simulink library "halout"  (R2021b)
settings: Solver=VariableStepAuto  StartTime=0.0  StopTime=10.0  RelTol=1e-3
undefined symbols (not defined in the file): C_TASK_5MS_S, KHAL_CAN1TxReq_flg, KHAL_CAN2TxReq_flg, KHAL_CAN3TxReq_flg, KHAL_CAN4TxReq_flg, KHAL_CAN5TxReq_flg, KHAL_CAN6TxReq_flg, KHAL_CAN7TxReq_flg, TRUE
libraries: FVT_lib x65, simulink x6
(part 4 of 6)

== system halout/HAL_OUT/CAN7/FD7_C100_0_0x19F005D0 ==
  BSCP_outputs : Inport  OutDataTypeStr=Bus: BSCP_outputs
  BOUTP_outputs : Inport  Port=2  OutDataTypeStr=Bus: BOUTP_outputs
  VCUKeyStatus : Subsystem
  bus_creator : BusCreator  Inputs=1  OutDataTypeStr=Bus: DT_CAN7_SG_FD7_C100_0  NonVirtualBus=on
  bus_selector : BusSelector  OutputSignals=VOUTP_Keystatus_enum
  FD7_C100_0 : Outport
  wires:
  BSCP_outputs/1 -> [BSCP_outputs]
  BOUTP_outputs/1 -> [BOUTP_outputs]
  [CAN7_VCUKeyStatus] -> bus_creator/1  "CAN7_VCUKeyStatus"
  bus_creator/1 -> FD7_C100_0/1
  VCUKeyStatus/1(CAN7_VCUKeyStatus) -> [CAN7_VCUKeyStatus]
  bus_selector/1 -> VCUKeyStatus/1(VCUKeyStatus)  "<VOUTP_Keystatus_enum>"
  [BOUTP_outputs] -> bus_selector/1

== system halout/HAL_OUT/CAN7/FD7_C10_0_0xC61D0D1 ==
  BSCP_outputs : Inport  OutDataTypeStr=Bus: BSCP_outputs
  BOUTP_outputs : Inport  Port=2  OutDataTypeStr=Bus: BOUTP_outputs
  EMotorSpd : Subsystem
  bus_creator : BusCreator  Inputs=1  OutDataTypeStr=Bus: DT_CAN7_SG_FD7_C10_0  NonVirtualBus=on
  bus_selector : BusSelector  OutputSignals=VOUTP_EVCU1EMotorSpd_rpm
  FD7_C10_0 : Outport
  wires:
  BSCP_outputs/1 -> [BSCP_outputs]
  BOUTP_outputs/1 -> [BOUTP_outputs]
  [CAN7_EMotorSpd] -> bus_creator/1  "CAN7_EMotorSpd"
  bus_creator/1 -> FD7_C10_0/1
  EMotorSpd/1(CAN7_EMotorSpd) -> [CAN7_EMotorSpd]
  bus_selector/1 -> EMotorSpd/1(EMotorSpd)  "<VOUTP_EVCU1EMotorSpd_rpm>"
  [BOUTP_outputs] -> bus_selector/1

== system halout/HAL_OUT/CAN7/FD7_C200_0_0x18F003EF ==
  BSCP_outputs : Inport  OutDataTypeStr=Bus: BSCP_outputs
  BOUTP_outputs : Inport  Port=2  OutDataTypeStr=Bus: BOUTP_outputs
  SysPowerMode : Subsystem
  bus_creator : BusCreator  Inputs=1  OutDataTypeStr=Bus: DT_CAN7_SG_FD7_C200_0  NonVirtualBus=on
  bus_selector : BusSelector  OutputSignals=VOUTP_SysPowerMode_enum
  FD7_C200_0 : Outport
  wires:
  BSCP_outputs/1 -> [BSCP_outputs]
  BOUTP_outputs/1 -> [BOUTP_outputs]
  [CAN7_SysPowerMode] -> bus_creator/1  "CAN7_SysPowerMode"
  bus_creator/1 -> FD7_C200_0/1
  SysPowerMode/1(CAN7_SysPowerMode) -> [CAN7_SysPowerMode]
  bus_selector/1 -> SysPowerMode/1(SysPowerMode)  "<VOUTP_SysPowerMode_enum>"
  [BOUTP_outputs] -> bus_selector/1

== system halout/HAL_OUT/CAN7/FD7_C50_0_0xCF00300 ==
  BSCP_outputs : Inport  OutDataTypeStr=Bus: BSCP_outputs
  BOUTP_outputs : Inport  Port=2  OutDataTypeStr=Bus: BOUTP_outputs
  AccPedalPos1 : Subsystem
  Ground : Ground
  bus_creator : BusCreator  Inputs=1  OutDataTypeStr=Bus: DT_CAN7_SG_FD7_C50_0  NonVirtualBus=on
  FD7_C50_0 : Outport
  wires:
  BSCP_outputs/1 -> [BSCP_outputs]
  BOUTP_outputs/1 -> [BOUTP_outputs]
  [CAN7_AccPedalPos1] -> bus_creator/1  "CAN7_AccPedalPos1"
  bus_creator/1 -> FD7_C50_0/1
  AccPedalPos1/1(CAN7_AccPedalPos1) -> [CAN7_AccPedalPos1]
  Ground/1 -> AccPedalPos1/1(AccPedalPos1)

== system halout/HAL_OUT/CAN7/FD7_CE100_0_0x18FA05B9 ==
  BSCP_outputs : Inport  OutDataTypeStr=Bus: BSCP_outputs
  BOUTP_outputs : Inport  Port=2  OutDataTypeStr=Bus: BOUTP_outputs
  FDCBCMDVRSignalLCmd : Subsystem
  FDCBCMDVRSignalRCmd : Subsystem
  FDCBCMFDoorSta : Subsystem
  FDCBCMHBeamCmd : Subsystem
  FDCBCMLBeamCmd : Subsystem
  FDCBCMMDoorSta : Subsystem
  FDCBCMPLampCmd : Subsystem
  bus_creator : BusCreator  Inputs=7  OutDataTypeStr=Bus: DT_CAN7_SG_FD7_CE100_0  NonVirtualBus=on
  bus_selector : BusSelector  OutputSignals=VOUTP_FDCBCMDVRSignalLCmd_flg
  bus_selector1 : BusSelector  OutputSignals=VOUTP_FDCBCMDVRSignalRCmd_flg
  bus_selector2 : BusSelector  OutputSignals=VOUTP_FDCBCMFDoorSta_flg
  bus_selector3 : BusSelector  OutputSignals=VOUTP_FDCBCMHBeamCmd_flg
  bus_selector4 : BusSelector  OutputSignals=VOUTP_FDCBCMLBeamCmd_flg
  bus_selector5 : BusSelector  OutputSignals=VOUTP_FDCBCMMDoorSta_flg
  bus_selector6 : BusSelector  OutputSignals=VOUTP_FDCBCMPLampCmd_flg
  FD7_CE100_0 : Outport
  wires:
  BSCP_outputs/1 -> [BSCP_outputs]
  BOUTP_outputs/1 -> [BOUTP_outputs]
  [CAN7_FDC_BCM_DVRSignalL_Cmd] -> bus_creator/1  "CAN7_FDC_BCM_DVRSignalL_Cmd"
  [CAN7_FDC_BCM_DVRSignalR_Cmd] -> bus_creator/2  "CAN7_FDC_BCM_DVRSignalR_Cmd"
  [CAN7_FDC_BCM_FDoor_Sta] -> bus_creator/3  "CAN7_FDC_BCM_FDoor_Sta"
  [CAN7_FDC_BCM_HBeam_Cmd] -> bus_creator/4  "CAN7_FDC_BCM_HBeam_Cmd"
  [CAN7_FDC_BCM_LBeam_Cmd] -> bus_creator/5  "CAN7_FDC_BCM_LBeam_Cmd"
  [CAN7_FDC_BCM_MDoor_Sta] -> bus_creator/6  "CAN7_FDC_BCM_MDoor_Sta"
  [CAN7_FDC_BCM_PLamp_Cmd] -> bus_creator/7  "CAN7_FDC_BCM_PLamp_Cmd"
  bus_creator/1 -> FD7_CE100_0/1
  FDCBCMDVRSignalLCmd/1(CAN7_FDC_BCM_DVRSignalL_Cmd) -> [CAN7_FDC_BCM_DVRSignalL_Cmd]
  FDCBCMDVRSignalRCmd/1(CAN7_FDC_BCM_DVRSignalR_Cmd) -> [CAN7_FDC_BCM_DVRSignalR_Cmd]
  FDCBCMFDoorSta/1(CAN7_FDC_BCM_FDoor_Sta) -> [CAN7_FDC_BCM_FDoor_Sta]
  FDCBCMHBeamCmd/1(CAN7_FDC_BCM_HBeam_Cmd) -> [CAN7_FDC_BCM_HBeam_Cmd]
  FDCBCMLBeamCmd/1(CAN7_FDC_BCM_LBeam_Cmd) -> [CAN7_FDC_BCM_LBeam_Cmd]
  FDCBCMMDoorSta/1(CAN7_FDC_BCM_MDoor_Sta) -> [CAN7_FDC_BCM_MDoor_Sta]
  FDCBCMPLampCmd/1(CAN7_FDC_BCM_PLamp_Cmd) -> [CAN7_FDC_BCM_PLamp_Cmd]
  bus_selector/1 -> FDCBCMDVRSignalLCmd/1(FDCBCMDVRSignalLCmd)  "<VOUTP_FDCBCMDVRSignalLCmd_flg>"
  [BOUTP_outputs] -> bus_selector/1
  bus_selector1/1 -> FDCBCMDVRSignalRCmd/1(FDCBCMDVRSignalRCmd)  "<VOUTP_FDCBCMDVRSignalRCmd_flg>"
  [BOUTP_outputs] -> bus_selector1/1
  bus_selector2/1 -> FDCBCMFDoorSta/1(FDCBCMFDoorSta)  "<VOUTP_FDCBCMFDoorSta_flg>"
  [BOUTP_outputs] -> bus_selector2/1
  bus_selector3/1 -> FDCBCMHBeamCmd/1(FDCBCMHBeamCmd)  "<VOUTP_FDCBCMHBeamCmd_flg>"
  [BOUTP_outputs] -> bus_selector3/1
  bus_selector4/1 -> FDCBCMLBeamCmd/1(FDCBCMLBeamCmd)  "<VOUTP_FDCBCMLBeamCmd_flg>"
  [BOUTP_outputs] -> bus_selector4/1
  bus_selector5/1 -> FDCBCMMDoorSta/1(FDCBCMMDoorSta)  "<VOUTP_FDCBCMMDoorSta_flg>"
  [BOUTP_outputs] -> bus_selector5/1
  bus_selector6/1 -> FDCBCMPLampCmd/1(FDCBCMPLampCmd)  "<VOUTP_FDCBCMPLampCmd_flg>"
  [BOUTP_outputs] -> bus_selector6/1

== system halout/HAL_OUT/CAN1/FD1_C100_0_0x18FE4A03/VCUEBSRd4BR ==
  VCUEBSRd4BR : Inport
  Data Type Conversion : DataTypeConversion  OutDataTypeStr=uint8  RndMeth=Round
  CAN1_VCUEBSRd4BR : Outport
  wires:
  Data Type Conversion/1 -> CAN1_VCUEBSRd4BR/1
  VCUEBSRd4BR/1 -> Data Type Conversion/1

== system halout/HAL_OUT/CAN1/FD1_C100_1_0x18FF602B/VCUEBSHBSw ==
  VCUEBSHBSw : Inport
  Data Type Conversion : DataTypeConversion  OutDataTypeStr=uint8  RndMeth=Round
  CAN1_VCUEBSHBSw : Outport
  wires:
  Data Type Conversion/1 -> CAN1_VCUEBSHBSw/1
  VCUEBSHBSw/1 -> Data Type Conversion/1

== system halout/HAL_OUT/CAN1/FD1_C100_1_0x18FF602B/VCUEBSHHSw ==
  VCUEBSHHSw : Inport
  Data Type Conversion : DataTypeConversion  OutDataTypeStr=uint8  RndMeth=Round
  CAN1_VCUEBSHHSw : Outport
  wires:
  Data Type Conversion/1 -> CAN1_VCUEBSHHSw/1
  VCUEBSHHSw/1 -> Data Type Conversion/1

== system halout/HAL_OUT/CAN1/FD1_C100_2_0x19F005D0/GearFlashInd ==
  GearFlashInd : Inport
  Data Type Conversion : DataTypeConversion  OutDataTypeStr=uint8  RndMeth=Round
  CAN1_GearFlashInd : Outport
  wires:
  Data Type Conversion/1 -> CAN1_GearFlashInd/1
  GearFlashInd/1 -> Data Type Conversion/1

== system halout/HAL_OUT/CAN1/FD1_C100_2_0x19F005D0/LVBattLow ==
  LVBattLow : Inport
  Data Type Conversion : DataTypeConversion  OutDataTypeStr=uint8  RndMeth=Round
  CAN1_LVBattLow : Outport
  wires:
  Data Type Conversion/1 -> CAN1_LVBattLow/1
  LVBattLow/1 -> Data Type Conversion/1

== system halout/HAL_OUT/CAN1/FD1_C100_2_0x19F005D0/PweLmtInd ==
  PweLmtInd : Inport
  Data Type Conversion : DataTypeConversion  OutDataTypeStr=uint8  RndMeth=Round
  CAN1_PweLmtInd : Outport
  wires:
  Data Type Conversion/1 -> CAN1_PweLmtInd/1
  PweLmtInd/1 -> Data Type Conversion/1

== system halout/HAL_OUT/CAN1/FD1_C100_2_0x19F005D0/VCUBCMBuzzReq ==
  VCUBCMBuzzReq : Inport
  Data Type Conversion : DataTypeConversion  OutDataTypeStr=uint8  RndMeth=Round
  CAN1_VCUBCMBuzzReq : Outport
  wires:
  Data Type Conversion/1 -> CAN1_VCUBCMBuzzReq/1
  VCUBCMBuzzReq/1 -> Data Type Conversion/1

== system halout/HAL_OUT/CAN1/FD1_C100_2_0x19F005D0/VCUDTCCurrCode ==
  VCUDTCCurrCode : Inport
  Data Type Conversion : DataTypeConversion  OutDataTypeStr=uint32  RndMeth=Round
  CAN1_VCUDTCCurrCode : Outport
  wires:
  Data Type Conversion/1 -> CAN1_VCUDTCCurrCode/1
  VCUDTCCurrCode/1 -> Data Type Conversion/1

== system halout/HAL_OUT/CAN1/FD1_C100_2_0x19F005D0/VCUDTCCurrSta ==
  VCUDTCCurrSta : Inport
  Data Type Conversion : DataTypeConversion  OutDataTypeStr=uint8  RndMeth=Round
  CAN1_VCUDTCCurrSta : Outport
  wires:
  Data Type Conversion/1 -> CAN1_VCUDTCCurrSta/1
  VCUDTCCurrSta/1 -> Data Type Conversion/1

== system halout/HAL_OUT/CAN1/FD1_C100_2_0x19F005D0/VCUDTCHisCode ==
  VCUDTCHisCode : Inport
  Data Type Conversion : DataTypeConversion  OutDataTypeStr=uint32  RndMeth=Round
  CAN1_VCUDTCHisCode : Outport
  wires:
  Data Type Conversion/1 -> CAN1_VCUDTCHisCode/1
  VCUDTCHisCode/1 -> Data Type Conversion/1

== system halout/HAL_OUT/CAN1/FD1_C100_2_0x19F005D0/VCUDTCHisSta ==
  VCUDTCHisSta : Inport
  Data Type Conversion : DataTypeConversion  OutDataTypeStr=uint8  RndMeth=Round
  CAN1_VCUDTCHisSta : Outport
  wires:
  Data Type Conversion/1 -> CAN1_VCUDTCHisSta/1
  VCUDTCHisSta/1 -> Data Type Conversion/1

== system halout/HAL_OUT/CAN1/FD1_C100_2_0x19F005D0/VCUKeyStatus ==
  VCUKeyStatus : Inport
  Data Type Conversion : DataTypeConversion  OutDataTypeStr=uint8  RndMeth=Round
  CAN1_VCUKeyStatus : Outport
  wires:
  Data Type Conversion/1 -> CAN1_VCUKeyStatus/1
  VCUKeyStatus/1 -> Data Type Conversion/1

== system halout/HAL_OUT/CAN1/FD1_C100_2_0x19F005D0/VCUWarnInd ==
  VCUWarnInd : Inport
  Data Type Conversion : DataTypeConversion  OutDataTypeStr=uint8  RndMeth=Round
  CAN1_VCUWarnInd : Outport
  wires:
  Data Type Conversion/1 -> CAN1_VCUWarnInd/1
  VCUWarnInd/1 -> Data Type Conversion/1

== system halout/HAL_OUT/CAN1/FD1_C100_2_0x19F005D0/VCUnoPBInd ==
  VCUnoPBInd : Inport
  Data Type Conversion : DataTypeConversion  OutDataTypeStr=uint8  RndMeth=Round
  CAN1_VCUnoPBInd : Outport
  wires:
  Data Type Conversion/1 -> CAN1_VCUnoPBInd/1
  VCUnoPBInd/1 -> Data Type Conversion/1

== system halout/HAL_OUT/CAN1/FD1_C100_3_0x18FEF100/BrakeSW ==
  BrakeSW : Inport
  Data Type Conversion : DataTypeConversion  OutDataTypeStr=uint8  RndMeth=Round
  CAN1_BrakeSW : Outport
  wires:
  Data Type Conversion/1 -> CAN1_BrakeSW/1
  BrakeSW/1 -> Data Type Conversion/1

== system halout/HAL_OUT/CAN1/FD1_C100_3_0x18FEF100/VCUVehSpd ==
  VCUVehSpd : Inport
  Data Type Conversion : DataTypeConversion  OutDataTypeStr=uint16  RndMeth=Round
  convert_out : FVT_lib/hal/convert_out  gain=0.00391  offset=0
  CAN1_VCUVehSpd : Outport
  wires:
  Data Type Conversion/1 -> CAN1_VCUVehSpd/1
  convert_out/1 -> Data Type Conversion/1
  VCUVehSpd/1 -> convert_out/1

== system halout/HAL_OUT/CAN1/FD1_C10_0_0xC61D0D1/VehActDriveDirect ==
  VehActDriveDirect : Inport
  Data Type Conversion : DataTypeConversion  OutDataTypeStr=uint8  RndMeth=Round
  CAN1_VehActDriveDirect : Outport
  wires:
  Data Type Conversion/1 -> CAN1_VehActDriveDirect/1
  VehActDriveDirect/1 -> Data Type Conversion/1

== system halout/HAL_OUT/CAN1/FD1_C10_1_0x18FF20EF/ActEMOutSftSpd ==
  ActEMOutSftSpd : Inport
  Data Type Conversion : DataTypeConversion  OutDataTypeStr=uint16  RndMeth=Round
  convert_out : FVT_lib/hal/convert_out  gain=0.25  offset=0
  CAN1_ActEMOutSftSpd : Outport
  wires:
  Data Type Conversion/1 -> CAN1_ActEMOutSftSpd/1
  convert_out/1 -> Data Type Conversion/1
  ActEMOutSftSpd/1 -> convert_out/1

== system halout/HAL_OUT/CAN1/FD1_C10_1_0x18FF20EF/ActEMpTrq ==
  ActEMpTrq : Inport
  Data Type Conversion : DataTypeConversion  OutDataTypeStr=uint8  RndMeth=Round
  convert_out : FVT_lib/hal/convert_out  gain=1  offset=-125
  CAN1_ActEMpTrq : Outport
  wires:
  Data Type Conversion/1 -> CAN1_ActEMpTrq/1
  convert_out/1 -> Data Type Conversion/1
  ActEMpTrq/1 -> convert_out/1

== system halout/HAL_OUT/CAN1/FD1_C10_1_0x18FF20EF/ActEMpTrqHrls ==
  ActEMpTrqHrls : Inport
  Data Type Conversion : DataTypeConversion  OutDataTypeStr=uint8  RndMeth=Round
  convert_out : FVT_lib/hal/convert_out  gain=0.125  offset=0
  CAN1_ActEMpTrqHrls : Outport
  wires:
  Data Type Conversion/1 -> CAN1_ActEMpTrqHrls/1
  convert_out/1 -> Data Type Conversion/1
  ActEMpTrqHrls/1 -> convert_out/1

== system halout/HAL_OUT/CAN1/FD1_C10_1_0x18FF20EF/ActMaxAvaEMRecpTrq ==
  ActMaxAvaEMRecpTrq : Inport
  Data Type Conversion : DataTypeConversion  OutDataTypeStr=uint8  RndMeth=Round
  convert_out : FVT_lib/hal/convert_out  gain=1  offset=-125
  CAN1_ActMaxAvaEMRecpTrq : Outport
  wires:
  Data Type Conversion/1 -> CAN1_ActMaxAvaEMRecpTrq/1
  convert_out/1 -> Data Type Conversion/1
  ActMaxAvaEMRecpTrq/1 -> convert_out/1

== system halout/HAL_OUT/CAN1/FD1_C10_1_0x18FF20EF/DrvDemEMRtapTrq ==
  DrvDemEMRtapTrq : Inport
  Data Type Conversion : DataTypeConversion  OutDataTypeStr=uint8  RndMeth=Round
  convert_out : FVT_lib/hal/convert_out  gain=1  offset=-125
  CAN1_DrvDemEMRtapTrq : Outport
  wires:
  Data Type Conversion/1 -> CAN1_DrvDemEMRtapTrq/1
  convert_out/1 -> Data Type Conversion/1
  DrvDemEMRtapTrq/1 -> convert_out/1

== system halout/HAL_OUT/CAN1/FD1_C10_1_0x18FF20EF/EMTrqModeDrvBrk ==
  EMTrqModeDrvBrk : Inport
  Data Type Conversion : DataTypeConversion  OutDataTypeStr=uint8  RndMeth=Round
  CAN1_EMTrqModeDrvBrk : Outport
  wires:
  Data Type Conversion/1 -> CAN1_EMTrqModeDrvBrk/1
  EMTrqModeDrvBrk/1 -> Data Type Conversion/1

== system halout/HAL_OUT/CAN1/FD1_C10_1_0x18FF20EF/RetSelNonEng ==
  RetSelNonEng : Inport
  Data Type Conversion : DataTypeConversion  OutDataTypeStr=uint8  RndMeth=Round
  convert_out : FVT_lib/hal/convert_out  gain=0.4  offset=0
  CAN1_RetSelNonEng : Outport
  wires:
  Data Type Conversion/1 -> CAN1_RetSelNonEng/1
  convert_out/1 -> Data Type Conversion/1
  RetSelNonEng/1 -> convert_out/1

== system halout/HAL_OUT/CAN1/FD1_C10_1_0x18FF20EF/SACtrlDev ==
  SACtrlDev : Inport
  Data Type Conversion : DataTypeConversion  OutDataTypeStr=uint8  RndMeth=Round
  CAN1_SACtrlDev : Outport
  wires:
  Data Type Conversion/1 -> CAN1_SACtrlDev/1
  SACtrlDev/1 -> Data Type Conversion/1

== system halout/HAL_OUT/CAN1/FD1_C200_0_0x18F003EF/SysPowerMode ==
  SysPowerMode : Inport
  Data Type Conversion : DataTypeConversion  OutDataTypeStr=uint8  RndMeth=Round
  CAN1_SysPowerMode : Outport
  wires:
  Data Type Conversion/1 -> CAN1_SysPowerMode/1
  SysPowerMode/1 -> Data Type Conversion/1

== system halout/HAL_OUT/CAN1/FD1_C20_0_0xC62D0D1/DCCurr ==
  DCCurr : Inport
  Data Type Conversion : DataTypeConversion  OutDataTypeStr=uint16  RndMeth=Round
  convert_out : FVT_lib/hal/convert_out  gain=0.05  offset=-1638.4
  CAN1_DCCurr : Outport
  wires:
  Data Type Conversion/1 -> CAN1_DCCurr/1
  convert_out/1 -> Data Type Conversion/1
  DCCurr/1 -> convert_out/1

== system halout/HAL_OUT/CAN1/FD1_C20_0_0xC62D0D1/DCVol ==
  DCVol : Inport
  Data Type Conversion : DataTypeConversion  OutDataTypeStr=uint16  RndMeth=Round
  convert_out : FVT_lib/hal/convert_out  gain=0.25  offset=0
  CAN1_DCVol : Outport
  wires:
  Data Type Conversion/1 -> CAN1_DCVol/1
  convert_out/1 -> Data Type Conversion/1
  DCVol/1 -> convert_out/1

== system halout/HAL_OUT/CAN1/FD1_C20_0_0xC62D0D1/MaxTorqAvail ==
  MaxTorqAvail : Inport
  Data Type Conversion : DataTypeConversion  OutDataTypeStr=uint16  RndMeth=Round
  convert_out : FVT_lib/hal/convert_out  gain=1  offset=-125
  CAN1_MaxTorqAvail : Outport
  wires:
  Data Type Conversion/1 -> CAN1_MaxTorqAvail/1
  convert_out/1 -> Data Type Conversion/1
  MaxTorqAvail/1 -> convert_out/1

== system halout/HAL_OUT/CAN1/FD1_C20_0_0xC62D0D1/MinTorqAvail ==
  MinTorqAvail : Inport
  Data Type Conversion : DataTypeConversion  OutDataTypeStr=uint16  RndMeth=Round
  convert_out : FVT_lib/hal/convert_out  gain=1  offset=-125
  CAN1_MinTorqAvail : Outport
  wires:
  Data Type Conversion/1 -> CAN1_MinTorqAvail/1
  convert_out/1 -> Data Type Conversion/1
  MinTorqAvail/1 -> convert_out/1

== system halout/HAL_OUT/CAN1/FD1_C250_0_0x18FEDFEF/EMParasLoss ==
  EMParasLoss : Inport
  Data Type Conversion : DataTypeConversion  OutDataTypeStr=uint8  RndMeth=Round
  convert_out : FVT_lib/hal/convert_out  gain=1  offset=-125
  CAN1_EMParasLoss : Outport
  wires:
  Data Type Conversion/1 -> CAN1_EMParasLoss/1
  convert_out/1 -> Data Type Conversion/1
  EMParasLoss/1 -> convert_out/1

== system halout/HAL_OUT/CAN1/FD1_C250_0_0x18FEDFEF/NFricPercTorq ==
  NFricPercTorq : Inport
  Data Type Conversion : DataTypeConversion  OutDataTypeStr=uint8  RndMeth=Round
  convert_out : FVT_lib/hal/convert_out  gain=1  offset=-125
  CAN1_NFricPercTorq : Outport
  wires:
  Data Type Conversion/1 -> CAN1_NFricPercTorq/1
  convert_out/1 -> Data Type Conversion/1
  NFricPercTorq/1 -> convert_out/1

== system halout/HAL_OUT/CAN1/FD1_C5000_0_0x18FEE1EF/RC1MaxRetSpdP2 ==
  RC1MaxRetSpdP2 : Inport
  Data Type Conversion : DataTypeConversion  OutDataTypeStr=uint16  RndMeth=Round
  convert_out : FVT_lib/hal/convert_out  gain=0.125  offset=0
  CAN1_RC1MaxRetSpdP2 : Outport
  wires:
  Data Type Conversion/1 -> CAN1_RC1MaxRetSpdP2/1
  convert_out/1 -> Data Type Conversion/1
  RC1MaxRetSpdP2/1 -> convert_out/1

== system halout/HAL_OUT/CAN1/FD1_C5000_0_0x18FEE1EF/RC1PctTrqIdleP1 ==
  RC1PctTrqIdleP1 : Inport
  Data Type Conversion : DataTypeConversion  OutDataTypeStr=uint8  RndMeth=Round
  convert_out : FVT_lib/hal/convert_out  gain=1  offset=-125
  CAN1_RC1PctTrqIdleP1 : Outport
  wires:
  Data Type Conversion/1 -> CAN1_RC1PctTrqIdleP1/1
  convert_out/1 -> Data Type Conversion/1
  RC1PctTrqIdleP1/1 -> convert_out/1

== system halout/HAL_OUT/CAN1/FD1_C5000_0_0x18FEE1EF/RC1PctTrqMaxSpdP2 ==
  RC1PctTrqMaxSpdP2 : Inport
  Data Type Conversion : DataTypeConversion  OutDataTypeStr=uint8  RndMeth=Round
  convert_out : FVT_lib/hal/convert_out  gain=1  offset=-125
  CAN1_RC1PctTrqMaxSpdP2 : Outport
  wires:
  Data Type Conversion/1 -> CAN1_RC1PctTrqMaxSpdP2/1
  convert_out/1 -> Data Type Conversion/1
  RC1PctTrqMaxSpdP2/1 -> convert_out/1

== system halout/HAL_OUT/CAN1/FD1_C5000_0_0x18FEE1EF/RC1PctTrqP3 ==
  RC1PctTrqP3 : Inport
  Data Type Conversion : DataTypeConversion  OutDataTypeStr=uint8  RndMeth=Round
  convert_out : FVT_lib/hal/convert_out  gain=1  offset=-125
  CAN1_RC1PctTrqP3 : Outport
  wires:
  Data Type Conversion/1 -> CAN1_RC1PctTrqP3/1
  convert_out/1 -> Data Type Conversion/1
  RC1PctTrqP3/1 -> convert_out/1

== system halout/HAL_OUT/CAN1/FD1_C5000_0_0x18FEE1EF/RC1PctTrqP4 ==
  RC1PctTrqP4 : Inport
  Data Type Conversion : DataTypeConversion  OutDataTypeStr=uint8  RndMeth=Round
  convert_out : FVT_lib/hal/convert_out  gain=1  offset=-125
  CAN1_RC1PctTrqP4 : Outport
  wires:
  Data Type Conversion/1 -> CAN1_RC1PctTrqP4/1
  convert_out/1 -> Data Type Conversion/1
  RC1PctTrqP4/1 -> convert_out/1

== system halout/HAL_OUT/CAN1/FD1_C5000_0_0x18FEE1EF/RC1PctTrqPekTrqP5 ==
  RC1PctTrqPekTrqP5 : Inport
  Data Type Conversion : DataTypeConversion  OutDataTypeStr=uint8  RndMeth=Round
  convert_out : FVT_lib/hal/convert_out  gain=1  offset=-125
  CAN1_RC1PctTrqPekTrqP5 : Outport
  wires:
  Data Type Conversion/1 -> CAN1_RC1PctTrqPekTrqP5/1
  convert_out/1 -> Data Type Conversion/1
  RC1PctTrqPekTrqP5/1 -> convert_out/1

== system halout/HAL_OUT/CAN1/FD1_C5000_0_0x18FEE1EF/RC1RefRetTrq ==
  RC1RefRetTrq : Inport
  Data Type Conversion : DataTypeConversion  OutDataTypeStr=uint16  RndMeth=Round
  CAN1_RC1RefRetTrq : Outport
  wires:
  Data Type Conversion/1 -> CAN1_RC1RefRetTrq/1
  RC1RefRetTrq/1 -> Data Type Conversion/1

== system halout/HAL_OUT/CAN1/FD1_C5000_0_0x18FEE1EF/RC1RetCtrlMth ==
  RC1RetCtrlMth : Inport
  Data Type Conversion : DataTypeConversion  OutDataTypeStr=uint8  RndMeth=Round
  convert_out : FVT_lib/hal/convert_out  gain=1  offset=-125
  CAN1_RC1RetCtrlMth : Outport
  wires:
  Data Type Conversion/1 -> CAN1_RC1RetCtrlMth/1
  convert_out/1 -> Data Type Conversion/1
  RC1RetCtrlMth/1 -> convert_out/1

== system halout/HAL_OUT/CAN1/FD1_C5000_0_0x18FEE1EF/RC1RetLocat ==
  RC1RetLocat : Inport
  Data Type Conversion : DataTypeConversion  OutDataTypeStr=uint8  RndMeth=Round
  CAN1_RC1RetLocat : Outport
  wires:
  Data Type Conversion/1 -> CAN1_RC1RetLocat/1
  RC1RetLocat/1 -> Data Type Conversion/1

== system halout/HAL_OUT/CAN1/FD1_C5000_0_0x18FEE1EF/RC1RetSpdIdleP1 ==
  RC1RetSpdIdleP1 : Inport
  Data Type Conversion : DataTypeConversion  OutDataTypeStr=uint16  RndMeth=Round
  convert_out : FVT_lib/hal/convert_out  gain=0.125  offset=0
  CAN1_RC1RetSpdIdleP1 : Outport
  wires:
  Data Type Conversion/1 -> CAN1_RC1RetSpdIdleP1/1
  convert_out/1 -> Data Type Conversion/1
  RC1RetSpdIdleP1/1 -> convert_out/1

== system halout/HAL_OUT/CAN1/FD1_C5000_0_0x18FEE1EF/RC1RetSpdP3 ==
  RC1RetSpdP3 : Inport
  Data Type Conversion : DataTypeConversion  OutDataTypeStr=uint16  RndMeth=Round
  convert_out : FVT_lib/hal/convert_out  gain=0.125  offset=0
  CAN1_RC1RetSpdP3 : Outport
  wires:
  Data Type Conversion/1 -> CAN1_RC1RetSpdP3/1
  convert_out/1 -> Data Type Conversion/1
  RC1RetSpdP3/1 -> convert_out/1

== system halout/HAL_OUT/CAN1/FD1_C5000_0_0x18FEE1EF/RC1RetSpdP4 ==
  RC1RetSpdP4 : Inport
  Data Type Conversion : DataTypeConversion  OutDataTypeStr=uint16  RndMeth=Round
  convert_out : FVT_lib/hal/convert_out  gain=0.125  offset=0
  CAN1_RC1RetSpdP4 : Outport
  wires:
  Data Type Conversion/1 -> CAN1_RC1RetSpdP4/1
  convert_out/1 -> Data Type Conversion/1
  RC1RetSpdP4/1 -> convert_out/1

== system halout/HAL_OUT/CAN1/FD1_C5000_0_0x18FEE1EF/RC1RetSpdPekTrqP5 ==
  RC1RetSpdPekTrqP5 : Inport
  Data Type Conversion : DataTypeConversion  OutDataTypeStr=uint16  RndMeth=Round
  CAN1_RC1RetSpdPekTrqP5 : Outport
  wires:
  Data Type Conversion/1 -> CAN1_RC1RetSpdPekTrqP5/1
  RC1RetSpdPekTrqP5/1 -> Data Type Conversion/1

== system halout/HAL_OUT/CAN1/FD1_C5000_0_0x18FEE1EF/RC1RetType ==
  RC1RetType : Inport
  Data Type Conversion : DataTypeConversion  OutDataTypeStr=uint8  RndMeth=Round
  CAN1_RC1RetType : Outport
  wires:
  Data Type Conversion/1 -> CAN1_RC1RetType/1
  RC1RetType/1 -> Data Type Conversion/1

== system halout/HAL_OUT/CAN1/FD1_C5000_1_0x18FEE3EF/EMDefTrqLmt ==
  EMDefTrqLmt : Inport
  Data Type Conversion : DataTypeConversion  OutDataTypeStr=uint16  RndMeth=Round
  convert_out : FVT_lib/hal/convert_out  gain=0.125  offset=0
  CAN1_EMDefTrqLmt : Outport
  wires:
  Data Type Conversion/1 -> CAN1_EMDefTrqLmt/1
  convert_out/1 -> Data Type Conversion/1
  EMDefTrqLmt/1 -> convert_out/1

== system halout/HAL_OUT/CAN1/FD1_C5000_1_0x18FEE3EF/EMEMRefTorq ==
  EMEMRefTorq : Inport
  Data Type Conversion : DataTypeConversion  OutDataTypeStr=uint16  RndMeth=Round
  CAN1_EMEMRefTorq : Outport
  wires:
  Data Type Conversion/1 -> CAN1_EMEMRefTorq/1
  EMEMRefTorq/1 -> Data Type Conversion/1

== system halout/HAL_OUT/CAN1/FD1_C5000_1_0x18FEE3EF/EMEMSpdP2 ==
  EMEMSpdP2 : Inport
  Data Type Conversion : DataTypeConversion  OutDataTypeStr=uint16  RndMeth=Round
  convert_out : FVT_lib/hal/convert_out  gain=0.125  offset=0
  CAN1_EMEMSpdP2 : Outport
  wires:
  Data Type Conversion/1 -> CAN1_EMEMSpdP2/1
  convert_out/1 -> Data Type Conversion/1
  EMEMSpdP2/1 -> convert_out/1

== system halout/HAL_OUT/CAN1/FD1_C5000_1_0x18FEE3EF/EMEMSpdP3 ==
  EMEMSpdP3 : Inport
  Data Type Conversion : DataTypeConversion  OutDataTypeStr=uint16  RndMeth=Round
  convert_out : FVT_lib/hal/convert_out  gain=0.125  offset=0
  CAN1_EMEMSpdP3 : Outport
  wires:
  Data Type Conversion/1 -> CAN1_EMEMSpdP3/1
  convert_out/1 -> Data Type Conversion/1
  EMEMSpdP3/1 -> convert_out/1

== system halout/HAL_OUT/CAN1/FD1_C5000_1_0x18FEE3EF/EMEMSpdP4 ==
  EMEMSpdP4 : Inport
  Data Type Conversion : DataTypeConversion  OutDataTypeStr=uint16  RndMeth=Round
  convert_out : FVT_lib/hal/convert_out  gain=0.125  offset=0
  CAN1_EMEMSpdP4 : Outport
  wires:
  Data Type Conversion/1 -> CAN1_EMEMSpdP4/1
  convert_out/1 -> Data Type Conversion/1
  EMEMSpdP4/1 -> convert_out/1

== system halout/HAL_OUT/CAN1/FD1_C5000_1_0x18FEE3EF/EMEMSpdP5 ==
  EMEMSpdP5 : Inport
  Data Type Conversion : DataTypeConversion  OutDataTypeStr=uint16  RndMeth=Round
  convert_out : FVT_lib/hal/convert_out  gain=0.125  offset=0
  CAN1_EMEMSpdP5 : Outport
  wires:
  Data Type Conversion/1 -> CAN1_EMEMSpdP5/1
  convert_out/1 -> Data Type Conversion/1
  EMEMSpdP5/1 -> convert_out/1

== system halout/HAL_OUT/CAN1/FD1_C5000_1_0x18FEE3EF/EMExtRSCtrlUpLmt ==
  EMExtRSCtrlUpLmt : Inport
  Data Type Conversion : DataTypeConversion  OutDataTypeStr=uint16  RndMeth=Round
  convert_out : FVT_lib/hal/convert_out  gain=0.125  offset=0
  CAN1_EMExtRSCtrlUpLmt : Outport
  wires:
  Data Type Conversion/1 -> CAN1_EMExtRSCtrlUpLmt/1
  convert_out/1 -> Data Type Conversion/1
  EMExtRSCtrlUpLmt/1 -> convert_out/1

== system halout/HAL_OUT/CAN1/FD1_C5000_1_0x18FEE3EF/EMGainEndSpdGvn ==
  EMGainEndSpdGvn : Inport
  Data Type Conversion : DataTypeConversion  OutDataTypeStr=uint16  RndMeth=Round
  convert_out : FVT_lib/hal/convert_out  gain=0.00078125  offset=0
  CAN1_EMGainEndSpdGvn : Outport
  wires:
  Data Type Conversion/1 -> CAN1_EMGainEndSpdGvn/1
  convert_out/1 -> Data Type Conversion/1
  EMGainEndSpdGvn/1 -> convert_out/1

== system halout/HAL_OUT/CAN1/FD1_C5000_1_0x18FEE3EF/EMMaxMEngOvrSP7 ==
  EMMaxMEngOvrSP7 : Inport
  Data Type Conversion : DataTypeConversion  OutDataTypeStr=uint16  RndMeth=Round
  convert_out : FVT_lib/hal/convert_out  gain=0.125  offset=0
  CAN1_EMMaxMEngOvrSP7 : Outport
  wires:
  Data Type Conversion/1 -> CAN1_EMMaxMEngOvrSP7/1
  convert_out/1 -> Data Type Conversion/1
  EMMaxMEngOvrSP7/1 -> convert_out/1

== system halout/HAL_OUT/CAN1/FD1_C5000_1_0x18FEE3EF/EMMaxMOvrTLmt ==
  EMMaxMOvrTLmt : Inport
  Data Type Conversion : DataTypeConversion  OutDataTypeStr=uint8  RndMeth=Round
  convert_out : FVT_lib/hal/convert_out  gain=0.1  offset=0
  CAN1_EMMaxMOvrTLmt : Outport
  wires:
  Data Type Conversion/1 -> CAN1_EMMaxMOvrTLmt/1
  convert_out/1 -> Data Type Conversion/1
  EMMaxMOvrTLmt/1 -> convert_out/1

== system halout/HAL_OUT/CAN1/FD1_C5000_1_0x18FEE3EF/EMMomOfInertia ==
  EMMomOfInertia : Inport
  Data Type Conversion : DataTypeConversion  OutDataTypeStr=uint16  RndMeth=Round
  convert_out : FVT_lib/hal/convert_out  gain=0.004  offset=0
  CAN1_EMMomOfInertia : Outport
  wires:
  Data Type Conversion/1 -> CAN1_EMMomOfInertia/1
  convert_out/1 -> Data Type Conversion/1
  EMMomOfInertia/1 -> convert_out/1

== system halout/HAL_OUT/CAN1/FD1_C5000_1_0x18FEE3EF/EMPercTorqIdleP1 ==
  EMPercTorqIdleP1 : Inport
  Data Type Conversion : DataTypeConversion  OutDataTypeStr=uint8  RndMeth=Round
  convert_out : FVT_lib/hal/convert_out  gain=1  offset=-125
  CAN1_EMPercTorqIdleP1 : Outport
  wires:
  Data Type Conversion/1 -> CAN1_EMPercTorqIdleP1/1
  convert_out/1 -> Data Type Conversion/1
  EMPercTorqIdleP1/1 -> convert_out/1

== system halout/HAL_OUT/CAN1/FD1_C5000_1_0x18FEE3EF/EMPercTorqP2 ==
  EMPercTorqP2 : Inport
  Data Type Conversion : DataTypeConversion  OutDataTypeStr=uint8  RndMeth=Round
  convert_out : FVT_lib/hal/convert_out  gain=1  offset=-125
  CAN1_EMPercTorqP2 : Outport
  wires:
  Data Type Conversion/1 -> CAN1_EMPercTorqP2/1
  convert_out/1 -> Data Type Conversion/1
  EMPercTorqP2/1 -> convert_out/1

== system halout/HAL_OUT/CAN1/FD1_C5000_1_0x18FEE3EF/EMPercTorqP3 ==
  EMPercTorqP3 : Inport
  Data Type Conversion : DataTypeConversion  OutDataTypeStr=uint8  RndMeth=Round
  convert_out : FVT_lib/hal/convert_out  gain=1  offset=-125
  CAN1_EMPercTorqP3 : Outport
  wires:
  Data Type Conversion/1 -> CAN1_EMPercTorqP3/1
  convert_out/1 -> Data Type Conversion/1
  EMPercTorqP3/1 -> convert_out/1

== system halout/HAL_OUT/CAN1/FD1_C5000_1_0x18FEE3EF/EMPercTorqP4 ==
  EMPercTorqP4 : Inport
  Data Type Conversion : DataTypeConversion  OutDataTypeStr=uint8  RndMeth=Round
  convert_out : FVT_lib/hal/convert_out  gain=1  offset=-125
  CAN1_EMPercTorqP4 : Outport
  wires:
  Data Type Conversion/1 -> CAN1_EMPercTorqP4/1
  convert_out/1 -> Data Type Conversion/1
  EMPercTorqP4/1 -> convert_out/1

== system halout/HAL_OUT/CAN1/FD1_C5000_1_0x18FEE3EF/EMPercTorqP5 ==
  EMPercTorqP5 : Inport
  Data Type Conversion : DataTypeConversion  OutDataTypeStr=uint8  RndMeth=Round
  convert_out : FVT_lib/hal/convert_out  gain=1  offset=-125
  CAN1_EMPercTorqP5 : Outport
  wires:
  Data Type Conversion/1 -> CAN1_EMPercTorqP5/1
  convert_out/1 -> Data Type Conversion/1
  EMPercTorqP5/1 -> convert_out/1

== system halout/HAL_OUT/CAN1/FD1_C5000_1_0x18FEE3EF/EMReqSpdCtrlLoLmt ==
  EMReqSpdCtrlLoLmt : Inport
  Data Type Conversion : DataTypeConversion  OutDataTypeStr=uint8  RndMeth=Round
  convert_out : FVT_lib/hal/convert_out  gain=10  offset=0
  CAN1_EMReqSpdCtrlLoLmt : Outport
  wires:
  Data Type Conversion/1 -> CAN1_EMReqSpdCtrlLoLmt/1
  convert_out/1 -> Data Type Conversion/1
  EMReqSpdCtrlLoLmt/1 -> convert_out/1

== system halout/HAL_OUT/CAN1/FD1_C5000_1_0x18FEE3EF/EMReqSpdCtrlUpLmt ==
  EMReqSpdCtrlUpLmt : Inport
  Data Type Conversion : DataTypeConversion  OutDataTypeStr=uint8  RndMeth=Round
  convert_out : FVT_lib/hal/convert_out  gain=10  offset=0
  CAN1_EMReqSpdCtrlUpLmt : Outport
  wires:
  Data Type Conversion/1 -> CAN1_EMReqSpdCtrlUpLmt/1
  convert_out/1 -> Data Type Conversion/1
  EMReqSpdCtrlUpLmt/1 -> convert_out/1

== system halout/HAL_OUT/CAN1/FD1_C5000_1_0x18FEE3EF/EMReqTrqCtrlLoLmt ==
  EMReqTrqCtrlLoLmt : Inport
  Data Type Conversion : DataTypeConversion  OutDataTypeStr=uint8  RndMeth=Round
  convert_out : FVT_lib/hal/convert_out  gain=1  offset=-125
  CAN1_EMReqTrqCtrlLoLmt : Outport
  wires:
  Data Type Conversion/1 -> CAN1_EMReqTrqCtrlLoLmt/1
  convert_out/1 -> Data Type Conversion/1
  EMReqTrqCtrlLoLmt/1 -> convert_out/1

== system halout/HAL_OUT/CAN1/FD1_C5000_1_0x18FEE3EF/EMReqTrqCtrlUpLmt ==
  EMReqTrqCtrlUpLmt : Inport
  Data Type Conversion : DataTypeConversion  OutDataTypeStr=uint8  RndMeth=Round
  convert_out : FVT_lib/hal/convert_out  gain=1  offset=-125
  CAN1_EMReqTrqCtrlUpLmt : Outport
  wires:
  Data Type Conversion/1 -> CAN1_EMReqTrqCtrlUpLmt/1
  convert_out/1 -> Data Type Conversion/1
  EMReqTrqCtrlUpLmt/1 -> convert_out/1

== system halout/HAL_OUT/CAN1/FD1_C5000_1_0x18FEE3EF/EMSpdHIdleP6 ==
  EMSpdHIdleP6 : Inport
  Data Type Conversion : DataTypeConversion  OutDataTypeStr=uint16  RndMeth=Round
  convert_out : FVT_lib/hal/convert_out  gain=0.125  offset=0
  CAN1_EMSpdHIdleP6 : Outport
  wires:
  Data Type Conversion/1 -> CAN1_EMSpdHIdleP6/1
  convert_out/1 -> Data Type Conversion/1
  EMSpdHIdleP6/1 -> convert_out/1

== system halout/HAL_OUT/CAN1/FD1_C5000_1_0x18FEE3EF/EMSpdIdleP1 ==
  EMSpdIdleP1 : Inport
  Data Type Conversion : DataTypeConversion  OutDataTypeStr=uint16  RndMeth=Round
  convert_out : FVT_lib/hal/convert_out  gain=0.125  offset=0
  CAN1_EMSpdIdleP1 : Outport
  wires:
  Data Type Conversion/1 -> CAN1_EMSpdIdleP1/1
  convert_out/1 -> Data Type Conversion/1
  EMSpdIdleP1/1 -> convert_out/1

== system halout/HAL_OUT/CAN1/FD1_C5000_1_0x18FEE3EF/EMSupTSC1CtrlPG1 ==
  EMSupTSC1CtrlPG1 : Inport
  Data Type Conversion : DataTypeConversion  OutDataTypeStr=uint8  RndMeth=Round
  CAN1_EMSupTSC1CtrlPG1 : Outport
  wires:
  Data Type Conversion/1 -> CAN1_EMSupTSC1CtrlPG1/1
  EMSupTSC1CtrlPG1/1 -> Data Type Conversion/1

== system halout/HAL_OUT/CAN1/FD1_C5000_1_0x18FEE3EF/EMSupTSC1CtrlPG2 ==
  EMSupTSC1CtrlPG2 : Inport
  Data Type Conversion : DataTypeConversion  OutDataTypeStr=uint8  RndMeth=Round
  CAN1_EMSupTSC1CtrlPG2 : Outport
  wires:
  Data Type Conversion/1 -> CAN1_EMSupTSC1CtrlPG2/1
  EMSupTSC1CtrlPG2/1 -> Data Type Conversion/1

== system halout/HAL_OUT/CAN1/FD1_C5000_1_0x18FEE3EF/EMSupTSC1CtrlPG3 ==
  EMSupTSC1CtrlPG3 : Inport
  Data Type Conversion : DataTypeConversion  OutDataTypeStr=uint8  RndMeth=Round
  CAN1_EMSupTSC1CtrlPG3 : Outport
  wires:
  Data Type Conversion/1 -> CAN1_EMSupTSC1CtrlPG3/1
  EMSupTSC1CtrlPG3/1 -> Data Type Conversion/1

== system halout/HAL_OUT/CAN1/FD1_C5000_1_0x18FEE3EF/EMSupTSC1CtrlPG4 ==
  EMSupTSC1CtrlPG4 : Inport
  Data Type Conversion : DataTypeConversion  OutDataTypeStr=uint8  RndMeth=Round
  CAN1_EMSupTSC1CtrlPG4 : Outport
  wires:
  Data Type Conversion/1 -> CAN1_EMSupTSC1CtrlPG4/1
  EMSupTSC1CtrlPG4/1 -> Data Type Conversion/1

== system halout/HAL_OUT/CAN1/FD1_C5000_1_0x18FEE3EF/EMSupVarRTSC1MSG ==
  EMSupVarRTSC1MSG : Inport
  Data Type Conversion : DataTypeConversion  OutDataTypeStr=uint8  RndMeth=Round
  CAN1_EMSupVarRTSC1MSG : Outport
  wires:
  Data Type Conversion/1 -> CAN1_EMSupVarRTSC1MSG/1
  EMSupVarRTSC1MSG/1 -> Data Type Conversion/1

== system halout/HAL_OUT/CAN1/FD1_C50_0_0x18F00503/ActDriveDirect ==
  ActDriveDirect : Inport
  Data Type Conversion : DataTypeConversion  OutDataTypeStr=uint8  RndMeth=Round
  convert_out : FVT_lib/hal/convert_out  gain=1  offset=-125
  CAN1_ActDriveDirect : Outport
  wires:
  Data Type Conversion/1 -> CAN1_ActDriveDirect/1
  convert_out/1 -> Data Type Conversion/1
  ActDriveDirect/1 -> convert_out/1

== system halout/HAL_OUT/CAN1/FD1_C50_1_0xCF00300/AccPedal1LowSW ==
  AccPedal1LowSW : Inport
  Data Type Conversion : DataTypeConversion  OutDataTypeStr=uint8  RndMeth=Round
  CAN1_AccPedal1LowSW : Outport
  wires:
  Data Type Conversion/1 -> CAN1_AccPedal1LowSW/1
  AccPedal1LowSW/1 -> Data Type Conversion/1

== system halout/HAL_OUT/CAN1/FD1_C50_1_0xCF00300/AccPedalPos1 ==
  AccPedalPos1 : Inport
  Data Type Conversion : DataTypeConversion  OutDataTypeStr=uint8  RndMeth=Round
  convert_out : FVT_lib/hal/convert_out  gain=0.4  offset=0
  CAN1_AccPedalPos1 : Outport
  wires:
  Data Type Conversion/1 -> CAN1_AccPedalPos1/1
  convert_out/1 -> Data Type Conversion/1
  AccPedalPos1/1 -> convert_out/1

== system halout/HAL_OUT/CAN1/FD1_C50_1_0xCF00300/EEC2MSGCS ==
  EEC2MSGCS : Inport
  Data Type Conversion : DataTypeConversion  OutDataTypeStr=uint8  RndMeth=Round
  CAN1_EEC2MSGCS : Outport
  wires:
  Data Type Conversion/1 -> CAN1_EEC2MSGCS/1
  EEC2MSGCS/1 -> Data Type Conversion/1

== system halout/HAL_OUT/CAN1/FD1_C50_1_0xCF00300/EEC2MSGCnt ==
  EEC2MSGCnt : Inport
  Data Type Conversion : DataTypeConversion  OutDataTypeStr=uint8  RndMeth=Round
  CAN1_EEC2MSGCnt : Outport
  wires:
  Data Type Conversion/1 -> CAN1_EEC2MSGCnt/1
  EEC2MSGCnt/1 -> Data Type Conversion/1

== system halout/HAL_OUT/CAN1/FD1_C80_0_0x18F00203/DLEngaged ==
  DLEngaged : Inport
  Data Type Conversion : DataTypeConversion  OutDataTypeStr=uint8  RndMeth=Round
  CAN1_DLEngaged : Outport
  wires:
  Data Type Conversion/1 -> CAN1_DLEngaged/1
  DLEngaged/1 -> Data Type Conversion/1

== system halout/HAL_OUT/CAN1/FD1_C80_0_0x18F00203/ShiftPgs ==
  ShiftPgs : Inport
  Data Type Conversion : DataTypeConversion  OutDataTypeStr=uint8  RndMeth=Round
  CAN1_ShiftPgs : Outport
  wires:
  Data Type Conversion/1 -> CAN1_ShiftPgs/1
  ShiftPgs/1 -> Data Type Conversion/1

== system halout/HAL_OUT/CAN1/FD1_CE100_0_0x18EBFFEF/CFGEM1DT0 ==
  CFGEM1DT0 : Inport
  Data Type Conversion : DataTypeConversion  OutDataTypeStr=uint8  RndMeth=Round
  CAN1_CFGEM1DT0 : Outport
  wires:
  Data Type Conversion/1 -> CAN1_CFGEM1DT0/1
  CFGEM1DT0/1 -> Data Type Conversion/1

== system halout/HAL_OUT/CAN1/FD1_CE100_0_0x18EBFFEF/CFGEM1DT1 ==
  CFGEM1DT1 : Inport
  Data Type Conversion : DataTypeConversion  OutDataTypeStr=uint8  RndMeth=Round
  CAN1_CFGEM1DT1 : Outport
  wires:
  Data Type Conversion/1 -> CAN1_CFGEM1DT1/1
  CFGEM1DT1/1 -> Data Type Conversion/1

== system halout/HAL_OUT/CAN1/FD1_CE100_0_0x18EBFFEF/CFGEM1DT2 ==
  CFGEM1DT2 : Inport
  Data Type Conversion : DataTypeConversion  OutDataTypeStr=uint8  RndMeth=Round
  CAN1_CFGEM1DT2 : Outport
  wires:
  Data Type Conversion/1 -> CAN1_CFGEM1DT2/1
  CFGEM1DT2/1 -> Data Type Conversion/1

== system halout/HAL_OUT/CAN1/FD1_CE100_0_0x18EBFFEF/CFGEM1DT3 ==
  CFGEM1DT3 : Inport
  Data Type Conversion : DataTypeConversion  OutDataTypeStr=uint8  RndMeth=Round
  CAN1_CFGEM1DT3 : Outport
  wires:
  Data Type Conversion/1 -> CAN1_CFGEM1DT3/1
  CFGEM1DT3/1 -> Data Type Conversion/1

== system halout/HAL_OUT/CAN1/FD1_CE100_0_0x18EBFFEF/CFGEM1DT4 ==
  CFGEM1DT4 : Inport
  Data Type Conversion : DataTypeConversion  OutDataTypeStr=uint8  RndMeth=Round
  CAN1_CFGEM1DT4 : Outport
  wires:
  Data Type Conversion/1 -> CAN1_CFGEM1DT4/1
  CFGEM1DT4/1 -> Data Type Conversion/1

== system halout/HAL_OUT/CAN1/FD1_CE100_0_0x18EBFFEF/CFGEM1DT5 ==
  CFGEM1DT5 : Inport
  Data Type Conversion : DataTypeConversion  OutDataTypeStr=uint8  RndMeth=Round
  CAN1_CFGEM1DT5 : Outport
  wires:
  Data Type Conversion/1 -> CAN1_CFGEM1DT5/1
  CFGEM1DT5/1 -> Data Type Conversion/1

== system halout/HAL_OUT/CAN1/FD1_CE100_0_0x18EBFFEF/CFGEM1DT6 ==
  CFGEM1DT6 : Inport
  Data Type Conversion : DataTypeConversion  OutDataTypeStr=uint8  RndMeth=Round
  CAN1_CFGEM1DT6 : Outport
  wires:
  Data Type Conversion/1 -> CAN1_CFGEM1DT6/1
  CFGEM1DT6/1 -> Data Type Conversion/1

== system halout/HAL_OUT/CAN1/FD1_CE100_0_0x18EBFFEF/CFGEM1DT7 ==
  CFGEM1DT7 : Inport
  Data Type Conversion : DataTypeConversion  OutDataTypeStr=uint8  RndMeth=Round
  CAN1_CFGEM1DT7 : Outport
  wires:
  Data Type Conversion/1 -> CAN1_CFGEM1DT7/1
  CFGEM1DT7/1 -> Data Type Conversion/1

== system halout/HAL_OUT/CAN1/FD1_CE100_1_0x18ECFFEF/CFGEM1BAMPGN ==
  CFGEM1BAMPGN : Inport
  Data Type Conversion : DataTypeConversion  OutDataTypeStr=uint32  RndMeth=Round
  CAN1_CFGEM1BAMPGN : Outport
  wires:
  Data Type Conversion/1 -> CAN1_CFGEM1BAMPGN/1
  CFGEM1BAMPGN/1 -> Data Type Conversion/1

== system halout/HAL_OUT/CAN1/FD1_CE100_1_0x18ECFFEF/CFGEM1BAMRsv ==
  CFGEM1BAMRsv : Inport
  Data Type Conversion : DataTypeConversion  OutDataTypeStr=uint8  RndMeth=Round
  CAN1_CFGEM1BAMRsv : Outport
  wires:
  Data Type Conversion/1 -> CAN1_CFGEM1BAMRsv/1
  CFGEM1BAMRsv/1 -> Data Type Conversion/1

== system halout/HAL_OUT/CAN1/FD1_CE100_1_0x18ECFFEF/CFGEM1BAMTNum ==
  CFGEM1BAMTNum : Inport
  Data Type Conversion : DataTypeConversion  OutDataTypeStr=uint8  RndMeth=Round
  CAN1_CFGEM1BAMTNum : Outport
  wires:
  Data Type Conversion/1 -> CAN1_CFGEM1BAMTNum/1
  CFGEM1BAMTNum/1 -> Data Type Conversion/1

== system halout/HAL_OUT/CAN1/FD1_CE100_1_0x18ECFFEF/CFGEM1BAMTSize ==
  CFGEM1BAMTSize : Inport
  Data Type Conversion : DataTypeConversion  OutDataTypeStr=uint16  RndMeth=Round
  CAN1_CFGEM1BAMTSize : Outport
  wires:
  Data Type Conversion/1 -> CAN1_CFGEM1BAMTSize/1
  CFGEM1BAMTSize/1 -> Data Type Conversion/1

== system halout/HAL_OUT/CAN1/FD1_CE100_1_0x18ECFFEF/CFGEM1Ctrl ==
  CFGEM1Ctrl : Inport
  Data Type Conversion : DataTypeConversion  OutDataTypeStr=uint8  RndMeth=Round
  CAN1_CFGEM1Ctrl : Outport
  wires:
  Data Type Conversion/1 -> CAN1_CFGEM1Ctrl/1
  CFGEM1Ctrl/1 -> Data Type Conversion/1

== system halout/HAL_OUT/CAN1/FD1_CE100_2_0x18FA05B9/FDCBCMDVRSignalLCmd ==
  FDCBCMDVRSignalLCmd : Inport
  Data Type Conversion : DataTypeConversion  OutDataTypeStr=uint8  RndMeth=Round
  CAN1_FDC_BCM_DVRSignalL_Cmd : Outport
  wires:
  Data Type Conversion/1 -> CAN1_FDC_BCM_DVRSignalL_Cmd/1
  FDCBCMDVRSignalLCmd/1 -> Data Type Conversion/1

== system halout/HAL_OUT/CAN1/FD1_CE100_2_0x18FA05B9/FDCBCMDVRSignalRCmd ==
  FDCBCMDVRSignalRCmd : Inport
  Data Type Conversion : DataTypeConversion  OutDataTypeStr=uint8  RndMeth=Round
  CAN1_FDC_BCM_DVRSignalR_Cmd : Outport
  wires:
  Data Type Conversion/1 -> CAN1_FDC_BCM_DVRSignalR_Cmd/1
  FDCBCMDVRSignalRCmd/1 -> Data Type Conversion/1

== system halout/HAL_OUT/CAN1/FD1_CE100_2_0x18FA05B9/FDCBCMLTurnLpCmd ==
  FDCBCMLTurnLpCmd : Inport
  Data Type Conversion : DataTypeConversion  OutDataTypeStr=uint8  RndMeth=Round
  CAN1_FDC_BCM_LTurnLp_Cmd : Outport
  wires:
  Data Type Conversion/1 -> CAN1_FDC_BCM_LTurnLp_Cmd/1
  FDCBCMLTurnLpCmd/1 -> Data Type Conversion/1

== system halout/HAL_OUT/CAN1/FD1_CE100_2_0x18FA05B9/FDCBCMRTurnLpCmd ==
  FDCBCMRTurnLpCmd : Inport
  Data Type Conversion : DataTypeConversion  OutDataTypeStr=uint8  RndMeth=Round
  CAN1_FDC_BCM_RTurnLp_Cmd : Outport
  wires:
  Data Type Conversion/1 -> CAN1_FDC_BCM_RTurnLp_Cmd/1
  FDCBCMRTurnLpCmd/1 -> Data Type Conversion/1

== system halout/HAL_OUT/CAN2/FD2_C1000_0_0x20E/VCUVehAcclLimit ==
  VCUVehAcclLimit : Inport
  Data Type Conversion : DataTypeConversion  OutDataTypeStr=uint8  RndMeth=Round
  convert_out : FVT_lib/hal/convert_out  gain=0.01  offset=0
  CAN2_VCUVehAcclLimit : Outport
  wires:
  Data Type Conversion/1 -> CAN2_VCUVehAcclLimit/1
  convert_out/1 -> Data Type Conversion/1
  VCUVehAcclLimit/1 -> convert_out/1

== system halout/HAL_OUT/CAN2/FD2_C1000_0_0x20E/VCUVehSpdlimit ==
  VCUVehSpdlimit : Inport
  Data Type Conversion : DataTypeConversion  OutDataTypeStr=uint8  RndMeth=Round
  CAN2_VCUVehSpdlimit : Outport
  wires:
  Data Type Conversion/1 -> CAN2_VCUVehSpdlimit/1
  VCUVehSpdlimit/1 -> Data Type Conversion/1

== system halout/HAL_OUT/CAN2/FD2_C10_0_0xC61D0D1/ActDriveMode ==
  ActDriveMode : Inport
  Data Type Conversion : DataTypeConversion  OutDataTypeStr=uint8  RndMeth=Round
  CAN2_ActDriveMode : Outport
  wires:
  Data Type Conversion/1 -> CAN2_ActDriveMode/1
  ActDriveMode/1 -> Data Type Conversion/1

== system halout/HAL_OUT/CAN2/FD2_C10_0_0xC61D0D1/CeTraxSysReady ==
  CeTraxSysReady : Inport
  Data Type Conversion : DataTypeConversion  OutDataTypeStr=uint8  RndMeth=Round
  CAN2_CeTraxSysReady : Outport
  wires:
  Data Type Conversion/1 -> CAN2_CeTraxSysReady/1
  CeTraxSysReady/1 -> Data Type Conversion/1

== system halout/HAL_OUT/CAN2/FD2_C10_0_0xC61D0D1/CreeperSta ==
  CreeperSta : Inport
  Data Type Conversion : DataTypeConversion  OutDataTypeStr=uint8  RndMeth=Round
  CAN2_CreeperSta : Outport
  wires:
  Data Type Conversion/1 -> CAN2_CreeperSta/1
  CreeperSta/1 -> Data Type Conversion/1

== system halout/HAL_OUT/CAN2/FD2_C10_0_0xC61D0D1/EBrakeTorqLow ==
  EBrakeTorqLow : Inport
  Data Type Conversion : DataTypeConversion  OutDataTypeStr=uint8  RndMeth=Round
  CAN2_EBrakeTorqLow : Outport
  wires:
  Data Type Conversion/1 -> CAN2_EBrakeTorqLow/1
  EBrakeTorqLow/1 -> Data Type Conversion/1

== system halout/HAL_OUT/CAN2/FD2_C10_0_0xC61D0D1/EMotorOverSpd ==
  EMotorOverSpd : Inport
  Data Type Conversion : DataTypeConversion  OutDataTypeStr=uint8  RndMeth=Round
  CAN2_EMotorOverSpd : Outport
  wires:
  Data Type Conversion/1 -> CAN2_EMotorOverSpd/1
  EMotorOverSpd/1 -> Data Type Conversion/1

== system halout/HAL_OUT/CAN2/FD2_C10_0_0xC61D0D1/EMotorPerformance ==
  EMotorPerformance : Inport
  Data Type Conversion : DataTypeConversion  OutDataTypeStr=uint16  RndMeth=Round
  convert_out : FVT_lib/hal/convert_out  gain=1  offset=-125
  CAN2_EMotorPerformance : Outport
  wires:
  Data Type Conversion/1 -> CAN2_EMotorPerformance/1
  convert_out/1 -> Data Type Conversion/1
  EMotorPerformance/1 -> convert_out/1

== system halout/HAL_OUT/CAN2/FD2_C10_0_0xC61D0D1/EMotorSpd ==
  EMotorSpd : Inport
  Data Type Conversion : DataTypeConversion  OutDataTypeStr=uint16  RndMeth=Round
  CAN2_EMotorSpd : Outport
  wires:
  Data Type Conversion/1 -> CAN2_EMotorSpd/1
  EMotorSpd/1 -> Data Type Conversion/1

== system halout/HAL_OUT/CAN2/FD2_C10_0_0xC61D0D1/EVECU1MSGCS ==
  EVECU1MSGCS : Inport
  Data Type Conversion : DataTypeConversion  OutDataTypeStr=uint8  RndMeth=Round
  CAN2_EVECU1MSGCS : Outport
  wires:
  Data Type Conversion/1 -> CAN2_EVECU1MSGCS/1
  EVECU1MSGCS/1 -> Data Type Conversion/1

== system halout/HAL_OUT/CAN2/FD2_C10_0_0xC61D0D1/EVECU1MSGCnt ==
  EVECU1MSGCnt : Inport
  Data Type Conversion : DataTypeConversion  OutDataTypeStr=uint8  RndMeth=Round
  CAN2_EVECU1MSGCnt : Outport
  wires:
  Data Type Conversion/1 -> CAN2_EVECU1MSGCnt/1
  EVECU1MSGCnt/1 -> Data Type Conversion/1

== system halout/HAL_OUT/CAN2/FD2_C10_0_0xC61D0D1/RecuperHighSta ==
  RecuperHighSta : Inport
  Data Type Conversion : DataTypeConversion  OutDataTypeStr=uint8  RndMeth=Round
  CAN2_RecuperHighSta : Outport
  wires:
  Data Type Conversion/1 -> CAN2_RecuperHighSta/1
  RecuperHighSta/1 -> Data Type Conversion/1

== system halout/HAL_OUT/CAN2/FD2_C10_0_0xC61D0D1/TUpASta ==
  TUpASta : Inport
  Data Type Conversion : DataTypeConversion  OutDataTypeStr=uint8  RndMeth=Round
  CAN2_TUpASta : Outport
  wires:
  Data Type Conversion/1 -> CAN2_TUpASta/1
  TUpASta/1 -> Data Type Conversion/1

== system halout/HAL_OUT/CAN2/FD2_C10_0_0xC61D0D1/VehActDriveDirect ==
  VehActDriveDirect : Inport
  Data Type Conversion : DataTypeConversion  OutDataTypeStr=uint8  RndMeth=Round
  CAN2_VehActDriveDirect : Outport
  wires:
  Data Type Conversion/1 -> CAN2_VehActDriveDirect/1
  VehActDriveDirect/1 -> Data Type Conversion/1

== system halout/HAL_OUT/CAN2/FD2_C10_0_0xC61D0D1/WheelSlipdet ==
  WheelSlipdet : Inport
  Data Type Conversion : DataTypeConversion  OutDataTypeStr=uint8  RndMeth=Round
  CAN2_WheelSlipdet : Outport
  wires:
  Data Type Conversion/1 -> CAN2_WheelSlipdet/1
  WheelSlipdet/1 -> Data Type Conversion/1

== system halout/HAL_OUT/CAN2/FD2_C200_0_0x20F/CACPresWarn ==
  CACPresWarn : Inport
  Data Type Conversion : DataTypeConversion  OutDataTypeStr=uint8  RndMeth=Round
  CAN2_CACPresWarn : Outport
  wires:
  Data Type Conversion/1 -> CAN2_CACPresWarn/1
  CACPresWarn/1 -> Data Type Conversion/1

== system halout/HAL_OUT/CAN2/FD2_C200_0_0x20F/FDCVCUVCUDRMSta ==
  FDCVCUVCUDRMSta : Inport
  Data Type Conversion : DataTypeConversion  OutDataTypeStr=uint8  RndMeth=Round
  CAN2_FDC_VCU_VCUDRM_Sta : Outport
  wires:
  Data Type Conversion/1 -> CAN2_FDC_VCU_VCUDRM_Sta/1
  FDCVCUVCUDRMSta/1 -> Data Type Conversion/1

== system halout/HAL_OUT/CAN2/FD2_C200_0_0x20F/SysPowerMode ==
  SysPowerMode : Inport
  Data Type Conversion : DataTypeConversion  OutDataTypeStr=uint8  RndMeth=Round
  CAN2_SysPowerMode : Outport
  wires:
  Data Type Conversion/1 -> CAN2_SysPowerMode/1
  SysPowerMode/1 -> Data Type Conversion/1

== system halout/HAL_OUT/CAN2/FD2_C500_0_0x18FA0517/IGNKeySta ==
  IGNKeySta : Inport
  Data Type Conversion : DataTypeConversion  OutDataTypeStr=uint8  RndMeth=Round
  CAN2_IGNKeySta : Outport
  wires:
  Data Type Conversion/1 -> CAN2_IGNKeySta/1
  IGNKeySta/1 -> Data Type Conversion/1

== system halout/HAL_OUT/CAN2/FD2_C500_0_0x18FA0517/VCUVehicleSpd ==
  VCUVehicleSpd : Inport
  Data Type Conversion : DataTypeConversion  OutDataTypeStr=uint16  RndMeth=Round
  convert_out : FVT_lib/hal/convert_out  gain=0.0039062  offset=0
  CAN2_VCU_VehicleSpd : Outport
  wires:
  Data Type Conversion/1 -> CAN2_VCU_VehicleSpd/1
  convert_out/1 -> Data Type Conversion/1
  VCUVehicleSpd/1 -> convert_out/1

== system halout/HAL_OUT/CAN2/FD2_C500_0_0x18FA0517/VSPFunc ==
  VSPFunc : Inport
  Data Type Conversion : DataTypeConversion  OutDataTypeStr=uint8  RndMeth=Round
  CAN2_VSPFunc : Outport
  wires:
  Data Type Conversion/1 -> CAN2_VSPFunc/1
  VSPFunc/1 -> Data Type Conversion/1

== system halout/HAL_OUT/CAN2/FD2_C50_0_0xCFF355A/EVEHCMSGCS ==
  EVEHCMSGCS : Inport
  Data Type Conversion : DataTypeConversion  OutDataTypeStr=uint8  RndMeth=Round
  CAN2_EVEHCMSGCS : Outport
  wires:
  Data Type Conversion/1 -> CAN2_EVEHCMSGCS/1
  EVEHCMSGCS/1 -> Data Type Conversion/1

== system halout/HAL_OUT/CAN2/FD2_C50_0_0xCFF355A/EVEHCMSGCnt ==
  EVEHCMSGCnt : Inport
  Data Type Conversion : DataTypeConversion  OutDataTypeStr=uint8  RndMeth=Round
  CAN2_EVEHCMSGCnt : Outport
  wires:
  Data Type Conversion/1 -> CAN2_EVEHCMSGCnt/1
  EVEHCMSGCnt/1 -> Data Type Conversion/1

== system halout/HAL_OUT/CAN2/FD2_C50_0_0xCFF355A/EVSysRls ==
  EVSysRls : Inport
  Data Type Conversion : DataTypeConversion  OutDataTypeStr=uint8  RndMeth=Round
  CAN2_EVSysRls : Outport
  wires:
  Data Type Conversion/1 -> CAN2_EVSysRls/1
  EVSysRls/1 -> Data Type Conversion/1

== system halout/HAL_OUT/CAN2/FD2_C50_0_0xCFF355A/ElecSysRdy ==
  ElecSysRdy : Inport
  Data Type Conversion : DataTypeConversion  OutDataTypeStr=uint8  RndMeth=Round
  CAN2_ElecSysRdy : Outport
  wires:
  Data Type Conversion/1 -> CAN2_ElecSysRdy/1
  ElecSysRdy/1 -> Data Type Conversion/1

== system halout/HAL_OUT/CAN2/FD2_C50_0_0xCFF355A/ExtAccLimReq ==
  ExtAccLimReq : Inport
  Data Type Conversion : DataTypeConversion  OutDataTypeStr=uint8  RndMeth=Round
  convert_out : FVT_lib/hal/convert_out  gain=0.01  offset=0
  CAN2_ExtAccLimReq : Outport
  wires:
  Data Type Conversion/1 -> CAN2_ExtAccLimReq/1
  convert_out/1 -> Data Type Conversion/1
  ExtAccLimReq/1 -> convert_out/1

== system halout/HAL_OUT/CAN2/FD2_C50_0_0xCFF355A/ExtDischgReq ==
  ExtDischgReq : Inport
  Data Type Conversion : DataTypeConversion  OutDataTypeStr=uint8  RndMeth=Round
  CAN2_ExtDischgReq : Outport
  wires:
  Data Type Conversion/1 -> CAN2_ExtDischgReq/1
  ExtDischgReq/1 -> Data Type Conversion/1

== system halout/HAL_OUT/CAN2/FD2_C50_0_0xCFF355A/ExtDriveMReq ==
  ExtDriveMReq : Inport
  Data Type Conversion : DataTypeConversion  OutDataTypeStr=uint8  RndMeth=Round
  CAN2_ExtDriveMReq : Outport
  wires:
  Data Type Conversion/1 -> CAN2_ExtDriveMReq/1
  ExtDriveMReq/1 -> Data Type Conversion/1

== system halout/HAL_OUT/CAN2/FD2_C50_0_0xCFF355A/ExtWorkshopMReq ==
  ExtWorkshopMReq : Inport
  Data Type Conversion : DataTypeConversion  OutDataTypeStr=uint8  RndMeth=Round
  CAN2_ExtWorkshopMReq : Outport
  wires:
  Data Type Conversion/1 -> CAN2_ExtWorkshopMReq/1
  ExtWorkshopMReq/1 -> Data Type Conversion/1

== system halout/HAL_OUT/CAN2/FD2_C50_0_0xCFF355A/RecuperLimOrReq ==
  RecuperLimOrReq : Inport
  Data Type Conversion : DataTypeConversion  OutDataTypeStr=uint8  RndMeth=Round
  CAN2_RecuperLimOrReq : Outport
  wires:
  Data Type Conversion/1 -> CAN2_RecuperLimOrReq/1
  RecuperLimOrReq/1 -> Data Type Conversion/1
